simulink model "dummy"  (R2018a)
settings: Solver=VariableStepAuto  StartTime=0.0  StopTime=10.0  RelTol=1e-3
settings Model: Creator=root  LastModifiedBy=root

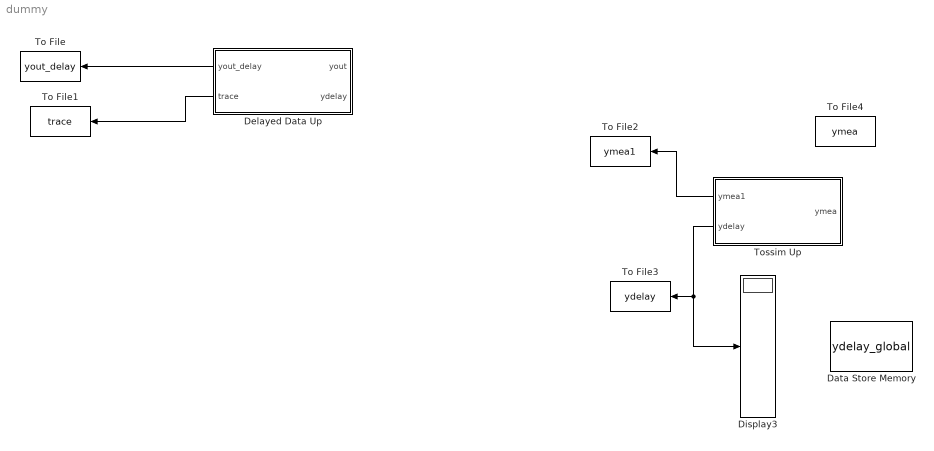
== system dummy ==
  Data Store Memory : DataStoreMemory  DataStoreName=ydelay_global  ReadBeforeWriteMsg=warning  WriteAfterWriteMsg=warning  WriteAfterReadMsg=warning  InitialValue=[1; 1; 1; 1; 1; 1; 1; 1; 1; 1; 1; 1; 1; 1; 1]  ShowAdditionalParam=off  OutDataTypeStr=uint32
  Delayed Data Up : MATLAB Function  TreatAsAtomicUnit=on
  Display3 : Display
  To File : ToFile  Filename=yout_delay  MatrixName=yout_delay1  SampleTime=1
  To File1 : ToFile  Filename=trace  MatrixName=trace1  SampleTime=1
  To File2 : ToFile  Filename=ymea1  MatrixName=ymea1  SampleTime=1
  To File3 : ToFile  Filename=ydelay  MatrixName=ydelay  SampleTime=1
  To File4 : ToFile  Filename=ymea  MatrixName=ymea  SampleTime=1
  Tossim Up : MATLAB Function  TreatAsAtomicUnit=on
  wires:
  Delayed Data Up/1(yout_delay) -> To File/1
  Delayed Data Up/2(trace) -> To File1/1
  Tossim Up/1(ymea1) -> To File2/1
  Tossim Up/2(ydelay) -> Display3/1, To File3/1

== matlab function dummy/Tossim Up ==
  data: ymea1 output; ymea input; ydelay output; ydelay_global data_store_memory
function [ymea1, ydelay]  = Tossim_block(ymea)
% Inputs:
% ymea: measurement from structure
% Outputs:
% ymea1: measurement output
% ydelay: delay traces
persistent delay1 past_ymea csi_ydelay% delay trace
persistent i  % count
global ydelay_global


% allow these matlab functions to be used in Embedded Matlab block
eml.extrinsic('python');
eml.extrinsic('num2str');
eml.extrinsic('str2num');
eml.extrinsic('delay_summary');
eml.extrinsic('disp');
eml.extrinsic('ps_aggregation');
eml.extrinsic('for');
eml.extrinsic('end');

if isempty(i)
    i = 0;
    %past_ymea = 0;
    past_ymea = ymea;
    csi_ydelay = past_ymea;
end

ydelay = [1 0 0 0 0 0 0 0 0]';
% call python to communicate with TOSSIM

call_count = 1; %Superframelength
rssi = -69;%sensor rssi

[resultz] = ps_aggregation(call_count, rssi);%here call TOSSIM Client ----yh
end_to_end_delivery_result_aggregated = sum(resultz)

resultz

[delay] = delay_summary(end_to_end_delivery_result_aggregated);

delay

ydelay = delay';

delay1 = ydelay;
x =ydelay(2);
i = i+1;

%ymea1 = ymea;

for i_yg = 1:9
    ydelay_global(i_yg, 1) = ydelay(i_yg, 1);
end
delay = ydelay';
for j=1:1
    if delay(1,j+1)~=88
        %csi_ydelay = past_ymea;
        ymea1 = past_ymea
        past_ymea = ymea
    else
        ymea1 = past_ymea
        ymea
    end
end

== matlab function dummy/Delayed Data Up ==
  data: yout input; ydelay input; yout_delay output; structure parameter; trace output
function [yout_delay,trace]   = delay_block(yout,ydelay, structure)

% Inputs: 
% yout: measurements output
% ydelay: delay traces
% structure: other necessary information 
% Inputs: 
% yout: measurements output
% ydelay: delay traces
% Outputs:
% yout_delay: delayed measurements output for controller

persistent  i yin_d 
persistent yin delay yin_all num past_y
eml.extrinsic('disp');

step_count=100000; %step_count

% initialize parameters
if isempty(yin)
    i = structure.i;
    yin = structure.yin; 
    yin_all = zeros(step_count+1,1); %zeros (step count, sensor number)    
    num = 0;
    past_y = 0;
end

num = num+1;   

%get delay information 
delay=ydelay';

%get value from "yout" input
for kk = 1:1
    yin_all(num,kk) = yout(kk);
end    
    
%generate output value according to delay    
for j=1:1
    if delay(1,j+1)~=88
        yin = yin_all(num,1);  %packet receive
        traces=1;
        past_y = yin;
    else
        yin=0;
        %yin = past_y;
        traces=0;        
    end
end

yin_d = yin';
yout_delay = yin_d;
trace=traces;

i = i+1;
